simulink model "Navion_6DoF_10_auto_ascend_2023"  (R2024a)
settings: Solver=ode45  StartTime=0.0  StopTime=500  FixedStep=.01  MaxStep=.004  RelTol=1e-5  EnableMultiTasking=on
values from neighbouring files (symbols this model uses):
  ac = [0 0 0]    [Navion_Geom_temp.m]
  b = 33.4    [Navion_Geom_temp.m]
  cbar = 5.7    [Navion_Geom_temp.m]
  cda2 = 0.33    [Navion_Geom_temp.m]
  cdo = 0.05    [Navion_Geom_temp.m]
  cg = [0 0 0]    [Navion_Geom_temp.m]
  cla = 4.44    [Navion_Geom_temp.m]
  cladot = 0    [Navion_Geom_temp.m]
  clb = -0.074    [Navion_Geom_temp.m]
  clda = -0.134    [Navion_Geom_temp.m]
  clde = 0.355    [Navion_Geom_temp.m]
  cldr = 0.107    [Navion_Geom_temp.m]
  clo = 0.41    [Navion_Geom_temp.m]
  clp = -0.410    (= -0.41)    [Navion_Geom_temp.m]
  clq = 3.8    [Navion_Geom_temp.m]
  clr = 0.107    [Navion_Geom_temp.m]
  cma = -0.683    [Navion_Geom_temp.m]
  cmadot = -4.36    [Navion_Geom_temp.m]
  cmde = -0.923    [Navion_Geom_temp.m]
  cmq = -9.96    [Navion_Geom_temp.m]
  cnb = 0.071    [Navion_Geom_temp.m]
  cnda = -0.0035    [Navion_Geom_temp.m]
  cndr = -0.072    [Navion_Geom_temp.m]
  cnp = -0.0575    [Navion_Geom_temp.m]
  cnr = -0.125    [Navion_Geom_temp.m]
  cyb = -0.564    [Navion_Geom_temp.m]
  cydr = 0.157    [Navion_Geom_temp.m]
  eng = [0 0 0]    [Navion_Geom_temp.m]
  initalt = 5000    [Navion_Geom_temp.m]
  initbank = 0    [Navion_Geom_temp.m]
  initeast = 0    [Navion_Geom_temp.m]
  inithead = 0    [Navion_Geom_temp.m]
  initnorth = 0    [Navion_Geom_temp.m]
  initp = 0    [Navion_Geom_temp.m]
  initpitch = initw/initu    (= 0)    [Navion_Geom_temp.m]
  initq = 0    [Navion_Geom_temp.m]
  initr = 0    [Navion_Geom_temp.m]
  initu = 223    [Navion_Geom_temp.m]
  initv = 0    [Navion_Geom_temp.m]
  initw = 0    [Navion_Geom_temp.m]
  jx = 1048    [Navion_Geom_temp.m]
  jxz = 0    [Navion_Geom_temp.m]
  jy = 3000    [Navion_Geom_temp.m]
  jz = 3500    [Navion_Geom_temp.m]
  sw = 184    [Navion_Geom_temp.m]
  weight = 2750    [Navion_Geom_temp.m]
undefined symbols (not defined in the file or in its folder): Earth, WGS84
libraries: simulink_extras x9, slpidlib x6, aerolibfltsims x2, simulink x2, aerolibtransform2 x1, aerolibanimutils x1
(part 1 of 2)
settings Model: Creator=andersop  LastModifiedBy=kaleb
settings SolverCC: InitialStep=.004  AlgebraicLoopSolver=TrustRegion
settings DataIOCC: LimitDataPoints=on  SaveFormat=Array  SignalLoggingSaveFormat=ModelDataLogs  SaveState=on  ReturnWorkspaceOutputs=off  SignalLoggingName=sigsOut
settings OptimizationCC: ExpressionDepthLimit=2147483647  InitFltsAndDblsToZero=on  LifeSpan=inf
settings DebuggingCC: SaveWithParameterizedLinksMsg=none  UnderspecifiedInitializationDetection=Classic  MergeDetectMultiDrivingBlocksExec=none  SignalResolutionControl=TryResolveAllWithWarning  MultiTaskDSMMsg=warning  MultiTaskCondExecSysMsg=none  FcnCallInpInsideContextMsg=warning  UnconnectedInputMsg=warning  UnconnectedOutputMsg=warning  UnconnectedLineMsg=warning  StateNameClashWarn=warning  SFUnexpectedBacktrackingDiag=warning  SFNoUnconditionalDefaultTransitionDiag=warning  SFExecutionAtInitializationDiag=none  ArithmeticOperatorsInVariantConditions=warning
settings HardwareCC: ProdBitPerPointer=32  ProdBitPerSizeT=32  ProdBitPerPtrDiffT=32  ProdLargestAtomicFloat=None  ProdIntDivRoundTo=Undefined  ProdEndianess=Unspecified  ProdWordSize=32  ProdHWDeviceType=32-bit Generic  TargetUnknown=on
settings ModelReferenceCC: PropagateSignalLabelsOutOfModel=off
settings SFSimCC: SimUseLocalCustomCode=off  CustomCodeUndefinedFunction=UseInterfaceOnly
settings RTWCC: RTWUseLocalCustomCode=off  GPUComputeCapability=3.5
settings CodeAppCC: StateflowObjectComments=on
settings GRTTargetCC: TargetFcnLib=ansi_tfl_tmw.mat  TargetLangStandard=C89/C90 (ANSI)  ModelReferenceCompliant=off  CombineOutputUpdateFcns=off  MatFileLogging=off  GRTInterface=on
settings ConfigComp: CovMetricSettings=dw  CovSaveCumulativeToWorkspaceVar=on  CovSaveSingleToWorkspaceVar=on  CovExternalEMLEnable=off

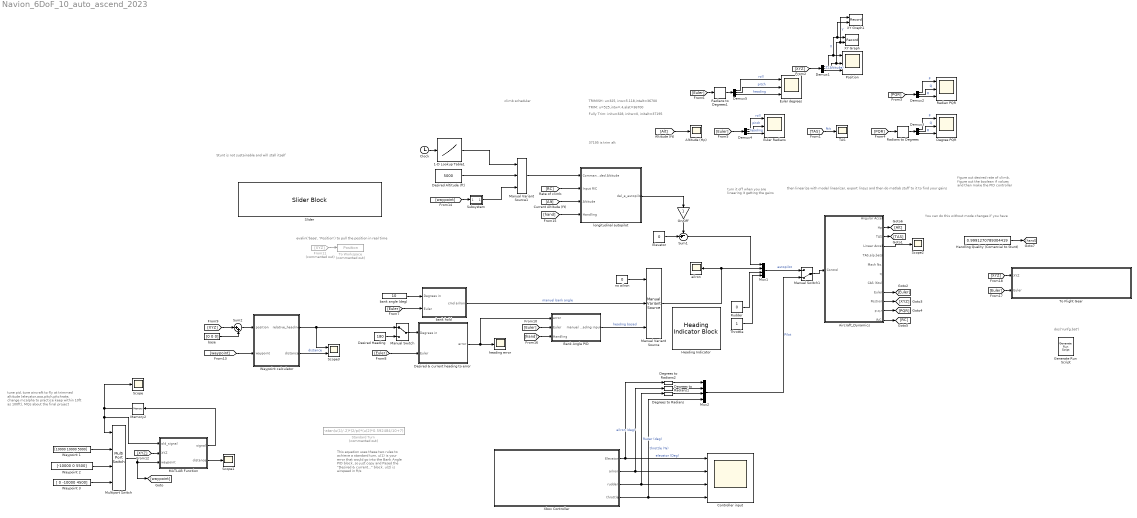
== system Navion_6DoF_10_auto_ascend_2023 ==
  note: tune pid, tune aircraft to fly at trimmed altitude (elevator,aoa,pitch,pitchrate, change mcalpha to practice keep within 10ft as 100ft), MQs about the final project
  note: Stunt is not sustainable and will stall itself
  note: This equation uses these two rules to achieve a standard turn, u(1) is your error that would go into the Bank Angle PID block, so just copy and Pased the "Desired & current..." block. u(2) is airspeed in ft/s
  note: evalin('base', 'Position') to pull the position in real time
  note: You can do this without mode changes if you have
  note: figure out desired rate of climb, figure out the boolean if values and then make the PID controller
  note: then linearize with model linearizer, export linsys and then do matlab stuff to it to find your gains
  note: turn it off when you are linearing it getting the gains
  note: climb scheduler
  note: 37195 is trim alt
  note: Fully Trim: initu=328, initw=0, initalt=37195
  note: TRIM: u=525,intw=.4,alat=36700
  note: TRIMISH: u=325, inw=5.118,intalt=36700
  note: dos('runfg.bat')
  1-D Lookup Table1 : Lookup_n-D  NumberOfTableDimensions=1  BreakpointsForDimension1=[0 50 51 400 401 800 801 900 901 1500]  Table=[37195;37195;34000;34000;37000;37000;30000;30000;31000;31000]  InternalRulePriority=Speed  RndMeth=Simplest
  Aircraft_Dynamics : Subsystem
  Altitude (Hp) : Scope
  Bank Angle PID : Subsystem
  Clock : Clock
  Controller input : Scope  NumInputPorts=4
  Degree PQR : Scope  NumInputPorts=3
  Degrees to Radians : simulink_extras/Transformations/Degrees to Radians
  Degrees to Radians1 : simulink_extras/Transformations/Degrees to Radians
  Degrees to Radians2 : simulink_extras/Transformations/Degrees to Radians
  Demux{1..5} (5 alike) : Demux  Outputs=3
  Desired & current heading to error : Subsystem
  Desired Altitude (ft) : Constant  Value=5000
  Desired Heading : Constant  Value=180
  Elevator : Constant  Value=0
  Euler Radians : Scope  NumInputPorts=3
  Euler degrees : Scope  NumInputPorts=3
  From11 : From  Commented=on  GotoTag=XYZ
  Generate Run Script : aerolibfltsims/Generate Run Script  Architecture=Win64  dataFlow=Send  GeometryModelName=c172p  AirportId=KSFO  RunwayId=01L  InitialAltitude=0  InitialHeading=0  OffsetDistance=0  OffsetAzimuth=0  InstallScenery=off  DisableShaders=on  OriginAddress=127.0.0.1  DestinationPort=5502  OriginPort=5505  LocalAddress=127.0.0.1  OutputFileName=runfg.bat  FlightGearBaseDirectory=C:\Program Files\FlightGear 2020.3
  Handling Quality (Comercial to Stunt) : Constant  Value=0.9991270789304419
  Heading Indicator : HeadingIndicatorBlock
  MATLAB Function : MATLAB Function  TreatAsAtomicUnit=on
  Manual Variant Source : simulink/Signal Routing/Manual Variant Source  NumChoices=3  LabelModeActiveChoice=V_3
  Manual Variant Source1 : simulink/Signal Routing/Manual Variant Source  NumChoices=3  LabelModeActiveChoice=V_3
  Manual Switch : ManualSwitch
  Manual Switch1 : ManualSwitch  CurrentSetting=0
  Memory2 : Memory  InitialCondition=1
  Multiport Switch : MultiPortSwitch  SaturateOnIntegerOverflow=off  InputSameDT=off
  Mux1 : Mux
  Mux2 : Mux
  On/Off : Gain
  Position : Scope  NumInputPorts=3
  Radian PQR : Scope  NumInputPorts=3
  Radians to Degrees : simulink_extras/Transformations/Radians to Degrees
  Radians to Degrees1 : simulink_extras/Transformations/Radians to Degrees
  Rudder : Constant  Value=0
  Scope : Scope
  Scope1 : Scope
  Scope2 : Scope
  Scope3 : Scope  NumInputPorts=2
  Slider : SliderBlock  ScaleMax=1
  Standard Turn : Fcn  Commented=on  Expr=-atan(u(1)/.2)*(2/pi)*(u(2)*0.592484/10+7)
  Subsystem : Subsystem
  Sum1 : Sum  Inputs=-+|
  Sum2 : Sum  Inputs=|++
  TAS : Scope
  Throttle : Constant
  To Flight Gear : Subsystem
  To Workspace : ToWorkspace  Commented=on  VariableName=Position  SaveFormat=Timeseries  SampleTime=-1
  Waypoint 1 : Constant  Value=[10000 10000 5000]
  Waypoint 2 : Constant  Value=[-10000 0 5500]
  Waypoint 3 : Constant  Value=[ 0 -10000 4500]
  Waypoint calculator : MATLAB Function  TreatAsAtomicUnit=on
  XY Graph : Record  FileSettingsInternal="{\"entries\":[{\"content\":{\"excelSettings\":{\"content\":{},\"type\":\"Streamout.ExcelSettings\"}},\"type\":\"Streamout.FileSettingStorage\",\"uuid\":\"\"}],\"packageUris\":[\"http:\\/\\/schema.mathworks.com\\/mf0\\/streamout_blocks\\/R2020a\"],\"version\":\"1.0\"}"  Layout=[1 1]  SignalsInternal="{\"entries\":[{\"content\":{\"signals\":[{\"content\":{\"blockPath\":[],\"dimensions\":[1],\"domain\":\"\",\"lineColor\":\"#a2142f\",\"lineWidth\":2,\"port\":1,\"sid\":[\"\"],\"signalID\":1,\"signalName\":\"X\"},\"type\":\"RecordBlkView.Signal\",\"uuid\":\"\"},{\"content\":{\"blockPath\":[],\"dimensions\":[1],\"domain\":\"\",\"lineColor\":\"#139fff\",\"lineWidth\":2,\"port\":2,\"sid\":[\"\"],\"signalID\":2,\"signalName\":\"Y\"},\"type\":\"RecordBlkView.Signal\",\"uuid\":\"\"}]},\"type\":\"RecordBlkView.InputSignals\",\"uuid\":\"\"}],\"packageUris\":[\"http:\\/\\/schema.mathworks.com\\/mf0\\/streamout_blocks\\/R2020a\"],\"version\":\"1.0\"}"  VisualizationBindings="{\"sparklinesplugin\":{\"info\":[{\"bindingParametersList\":[],\"subplotID\":1}]}}"  CompatibilityTag=XY
  XY Graph1 : Record  FileSettingsInternal="{\"entries\":[{\"content\":{\"excelSettings\":{\"content\":{},\"type\":\"Streamout.ExcelSettings\"}},\"type\":\"Streamout.FileSettingStorage\",\"uuid\":\"\"}],\"packageUris\":[\"http:\\/\\/schema.mathworks.com\\/mf0\\/streamout_blocks\\/R2020a\"],\"version\":\"1.0\"}"  Layout=[1 1]  SignalsInternal="{\"entries\":[{\"content\":{\"signals\":[{\"content\":{\"blockPath\":[],\"dimensions\":[1],\"domain\":\"\",\"lineColor\":\"#a2142f\",\"plots\":[ 1 ],\"port\":1,\"sid\":[\"\"],\"signalID\":1,\"signalName\":\"Y\"},\"type\":\"RecordBlkView.Signal\",\"uuid\":\"\"},{\"content\":{\"blockPath\":[],\"dimensions\":[1],\"domain\":\"\",\"lineColor\":\"#139fff\",\"plots\":[ 1 ],\"port\":2,\"sid\":[\"\"],\"signalID\":2,\"signalName\":\"X\"},\"type\":\"RecordBlkView.Signal\",\"uuid\":\"\"}]},\"type\":\"RecordBlkView.InputSignals\",\"uuid\":\"\"}],\"packageUris\":[\"http:\\/\\/schema.mathworks.com\\/mf0\\/streamout_blocks\\/R2020a\"],\"version\":\"1.0\"}"  VisualizationBindings="{\"xyplotplugin\":{\"info\":[{\"series\":[{\"bindingParametersList\":[{\"parameter\":\"X-Axis\",\"signalID\":1,\"signalName\":\"Y\"},{\"parameter\":\"Y-Axis\",\"signalID\":2,\"signalName\":\"X\"}],\"seriesID\":0}],\"subplotID\":1}]}}"  CompatibilityTag=XY
  Xbox Controller : Subsystem
  ailron : Scope
  bank angle (deg) : Constant  Value=10
  bank hold : Subsystem
  base : Constant  Value=[0 0 0]
  heading error : Scope
  longitudinal autopilot : Subsystem
  no ailron : Constant  Value=0
  wires:
  Elevator/1 -> Sum1/2
  Throttle/1 -> Mux1/4
  Mux1/1 -> Manual Switch1/1  "autopilot"
  Aircraft_Dynamics/2(Hp) -> [Alt]
  Aircraft_Dynamics/3(TAS) -> [TAS]
  Aircraft_Dynamics/9(Euler) -> [Euler]
  Aircraft_Dynamics/10(Postion) -> [XYZ]
  Aircraft_Dynamics/11(p,q,r) -> [PQR]
  [TAS] -> TAS/1  "ft/s"
  Demux1/3 -> Position/3  "Z (Altitude)"
  Demux1/2 -> XY Graph1/1, XY Graph/2, Position/2  "Y"
  Demux1/1 -> XY Graph1/2, XY Graph/1, Position/1  "X"
  [XYZ] -> Demux1/1
  [PQR] -> Demux2/1
  Demux2/1 -> Radian PQR/1  "P"
  Demux2/2 -> Radian PQR/2  "Q"
  Demux2/3 -> Radian PQR/3  "R"
  Demux3/3 -> Degree PQR/3  "R"
  Demux3/2 -> Degree PQR/2  "Q"
  Demux3/1 -> Degree PQR/1  "P"
  [PQR] -> Radians to Degrees/1
  Radians to Degrees/1 -> Demux3/1
  [Euler] -> Demux4/1
  Demux4/1 -> Euler Radians/1  "roll"
  Demux4/2 -> Euler Radians/2  "pitch"
  Demux4/3 -> Euler Radians/3  "heading"
  Demux5/3 -> Euler degrees/3  "heading"
  Demux5/2 -> Euler degrees/2  "pitch"
  Demux5/1 -> Euler degrees/1  "roll"
  [Euler] -> Radians to Degrees1/1
  Radians to Degrees1/1 -> Demux5/1
  Sum1/1 -> Mux1/1
  On/Off/1 -> Sum1/1
  [Alt] -> Altitude (Hp)/1
  longitudinal autopilot/1(del_e_autopilot) -> On/Off/1
  Desired Altitude (ft)/1 -> Manual Variant Source1/2
  [Alt] -> longitudinal autopilot/3(Altitude)
  Aircraft_Dynamics/12(R/C) -> [RC]
  [RC] -> longitudinal autopilot/2(Input R/C)
  Clock/1 -> 1-D Lookup Table1/1
  Rudder/1 -> Mux1/3
  [XYZ] -> Sum2/1
  Waypoint calculator/2(distance) -> Scope3/2  "distance"
  Waypoint calculator/1(relative_heading) -> Manual Switch/1, Scope3/1
  Desired Heading/1 -> Manual Switch/2
  Manual Variant Source/1 -> Mux1/2, ailron/1
  bank angle (deg)/1 -> bank hold/1(Degrees in)
  bank hold/1(cmd ailron) -> Manual Variant Source/2  "manuel bank angle"
  no ailron/1 -> Manual Variant Source/1
  [Euler] -> Desired & current heading to error/2(Euler)
  [Euler] -> bank hold/2(Euler)
  Desired & current heading to error/1(error) -> Bank Angle PID/1(error), heading error/1
  [Euler] -> Bank Angle PID/2(Euler)
  Bank Angle PID/1(manuel heading input) -> Manual Variant Source/3  "heading based"
  Waypoint 1/1 -> Multiport Switch/2
  Waypoint 2/1 -> Multiport Switch/3
  Waypoint 3/1 -> Multiport Switch/4
  Sum2/1 -> Waypoint calculator/1(position)
  base/1 -> Sum2/2
  From11/1 -> To Workspace/1
  Manual Switch/1 -> Desired & current heading to error/1(Degrees in)
  Multiport Switch/1 -> [waypoint], MATLAB Function/3(waypoint)
  [XYZ] -> MATLAB Function/2(XYZ)
  MATLAB Function/1(signal) -> Memory2/1
  Memory2/1 -> Multiport Switch/1, MATLAB Function/1(old_signal), Scope/1
  [waypoint] -> Waypoint calculator/2(waypoint)
  Manual Variant Source1/1 -> longitudinal autopilot/1(Commanded Altitude)
  1-D Lookup Table1/1 -> Manual Variant Source1/1
  [waypoint] -> Subsystem/1(In1)
  Subsystem/1(Out1) -> Manual Variant Source1/3
  MATLAB Function/2(distance) -> Scope1/1
  Aircraft_Dynamics/4(Linear Accel) -> Scope2/1
  Handling Quality (Comercial to Stunt)/1 -> [hand]
  [hand] -> longitudinal autopilot/4(Handling)
  [hand] -> Bank Angle PID/3(Handling)
  Xbox Controller/2(ailron) -> Degrees to Radians1/1, Controller input/2  "ailron (deg)"
  Xbox Controller/1(Elevator) -> Degrees to Radians2/1, Controller input/1  "elevator (Deg)"
  Xbox Controller/3(rudder) -> Degrees to Radians/1, Controller input/3  "Ruder (deg)"
  Xbox Controller/4(throttle) -> Mux2/4, Controller input/4  "throttle (%)"
  Degrees to Radians/1 -> Mux2/3
  Degrees to Radians2/1 -> Mux2/1
  Degrees to Radians1/1 -> Mux2/2
  Manual Switch1/1 -> Aircraft_Dynamics/1(Control)
  Mux2/1 -> Manual Switch1/2  "Pilot"
  [XYZ] -> To Flight Gear/1(XYZ)
  [Euler] -> To Flight Gear/2(Euler)

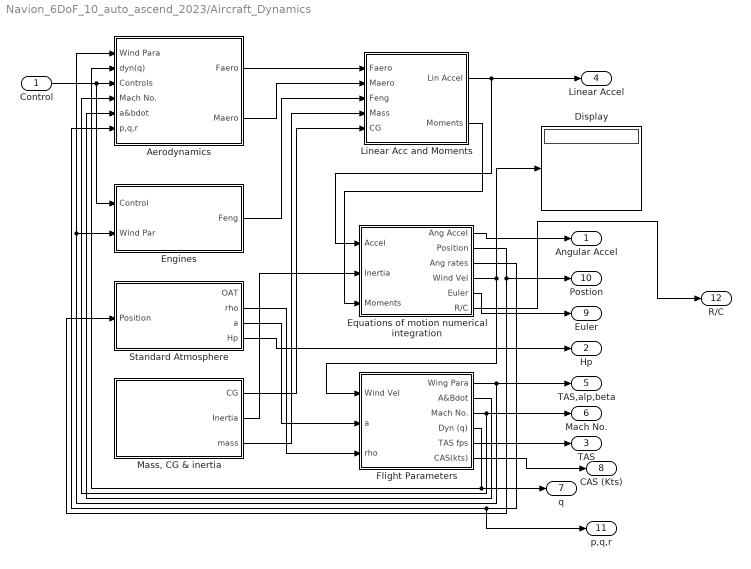
== system Navion_6DoF_10_auto_ascend_2023/Aircraft_Dynamics ==
  Control : Inport
  Aerodynamics : Subsystem
  Display : Display
  Engines : Subsystem
  "Equations of motion numerical integration " : Subsystem
  Flight Parameters : Subsystem
  Linear Acc and Moments : Subsystem
  "Mass, CG & inertia" : Subsystem
  Standard Atmosphere : Subsystem
  Angular Accel : Outport
  Hp : Outport  Port=2
  TAS : Outport  Port=3
  Linear Accel : Outport  Port=4
  TAS,alp,beta : Outport  Port=5
  Mach No. : Outport  Port=6
  q : Outport  Port=7
  CAS (Kts) : Outport  Port=8
  Euler : Outport  Port=9
  Postion : Outport  Port=10
  p,q,r : Outport  Port=11
  R/C : Outport  Port=12
  wires:
  Aerodynamics/1(Faero) -> Linear Acc and Moments/1(Faero)
  Aerodynamics/2(Maero) -> Linear Acc and Moments/2(Maero)
  Control/1 -> Aerodynamics/3(Controls), Engines/1(Control)
  Engines/1(Feng) -> Linear Acc and Moments/3(Feng)
  "Mass, CG & inertia"/1(CG) -> Linear Acc and Moments/5(CG)
  "Mass, CG & inertia"/2(Inertia) -> "Equations of motion numerical integration "/2(Inertia)
  Linear Acc and Moments/1(Lin Accel) -> "Equations of motion numerical integration "/1(Accel), Linear Accel/1
  Linear Acc and Moments/2(Moments) -> "Equations of motion numerical integration "/3(Moments)
  "Equations of motion numerical integration "/3(Ang rates) -> Aerodynamics/6(p,q,r), p,q,r/1
  "Equations of motion numerical integration "/4(Wind Vel) -> Flight Parameters/1(Wind Vel), Display/1
  Flight Parameters/1(Wing Para) -> TAS,alp,beta/1, Aerodynamics/1(Wind Para), Engines/2(Wind Par)
  Flight Parameters/4(Dyn (q)) -> Aerodynamics/2(dyn(q)), q/1
  Flight Parameters/3(Mach No.) -> Mach No./1, Aerodynamics/4(Mach No.)
  Flight Parameters/2(A&Bdot) -> Aerodynamics/5(a&bdot)
  "Equations of motion numerical integration "/2(Position) -> Postion/1, Standard Atmosphere/1(Position)
  "Equations of motion numerical integration "/1(Ang Accel) -> Angular Accel/1
  Standard Atmosphere/4(Hp) -> Hp/1
  Flight Parameters/5(TAS fps) -> TAS/1
  Flight Parameters/6(CAS(kts)) -> CAS (Kts)/1
  "Equations of motion numerical integration "/5(Euler) -> Euler/1
  Standard Atmosphere/3(a) -> Flight Parameters/2(a)
  Standard Atmosphere/2(rho) -> Flight Parameters/3(rho)
  "Mass, CG & inertia"/3(mass) -> Linear Acc and Moments/4(Mass)
  "Equations of motion numerical integration "/6(R/C) -> R/C/1

== system Navion_6DoF_10_auto_ascend_2023/Bank Angle PID ==
  note: agressive, will make it
  note: safe, wont make it
  note: was 50/23
  error : Inport
  Euler : Inport  Port=2
  Handling : Inport  Port=3
  Mux : Mux  Inputs=2
  PID Controller : slpidlib/PID Controller  Controller=PID  Form=Parallel  TimeDomain=Continuous-time  UseExternalTs=off  SampleTime=-1  IntegratorMethod=Forward Euler  FilterMethod=Forward Euler  ControllerParametersSource=internal  P=-0.426657604109643  I=-0.0814157073414658  UseKiTs=off  D=0.00186667465731567  UseExternalDerivativeSource=off  N=228.565595208321  UseFilter=on  TunerSelectOption=Transfer Function Based (PID Tuner App)  InitialConditionSource=internal  InitialConditionForIntegrator=0  InitialConditionForFilter=0  DifferentiatorICPrevScaledInput=0  ExternalReset=none  TrackingMode=off  Kt=1  LimitOutput=on  SatLimitsSource=internal  UpperSaturationLimit=.5  LowerSaturationLimit=-.5  LinearizeAsGain=off  AntiWindupMode=none  Kb=1  LimitIntegrator=off  UpperIntegratorSaturationLimit=inf  LowerIntegratorSaturationLimit=-inf  POutMin=[]  POutMax=[]  IOutMin=[]  IOutMax=[]  DOutMin=[]  DOutMax=[]  NOutMin=[]  NOutMax=[]  SumOutMin=[]  SumOutMax=[]  SaturationOutMin=[]  SaturationOutMax=[]  PParamMin=[]  PParamMax=[]  IParamMin=[]  IParamMax=[]  DParamMin=[]  DParamMax=[]  NParamMin=[]  NParamMax=[]  KbParamMin=[]  KbParamMax=[]  KtParamMin=[]  KtParamMax=[]  KbOutMin=[]  KbOutMax=[]  KtOutMin=[]  KtOutMax=[]  IntegratorOutMin=[]  IntegratorOutMax=[]  FilterOutMin=[]  FilterOutMax=[]  SumI1OutMin=[]  SumI1OutMax=[]  SumI2OutMin=[]  SumI2OutMax=[]  SumI3OutMin=[]  SumI3OutMax=[]  SumI4OutMin=[]  SumI4OutMax=[]  SumDOutMin=[]  SumDOutMax=[]  DifferentiatorOutMin=[]  DifferentiatorOutMax=[]  FilterDiffOutCoefMin=[]  FilterDiffOutCoefMax=[]  ReciprocalOutMin=[]  ReciprocalOutMax=[]  SumDenOutMin=[]  SumDenOutMax=[]  SumNumOutMin=[]  SumNumOutMax=[]  DivideOutMin=[]  DivideOutMax=[]  UdiffTsProdOutMin=[]  UdiffTsProdOutMax=[]  NTsProdOutMin=[]  NTsProdOutMax=[]  UintegralTsProdOutMin=[]  UintegralTsProdOutMax=[]  UngainTsProdOutMin=[]  UngainTsProdOutMax=[]  ClampingZeroOutDataTypeStr=Inherit: Inherit via back propagation  ClampingZeroOutMin=[]  ClampingZeroOutMax=[]  FilterDenConstantOutDataTypeStr=Inherit: Inherit via back propagation  FilterDenConstantOutMin=[]  FilterDenConstantOutMax=[]  PCopyOutDataTypeStr=Inherit: Inherit via back propagation  PCopyOutMin=[]  PCopyOutMax=[]  NCopyOutDataTypeStr=Inherit: Inherit via back propagation  NCopyOutMin=[]  NCopyOutMax=[]  IntegratorContinuousStateAttributes=''  IntegratorStateMustResolveToSignalObject=off  IntegratorRTWStateStorageClass=Auto  FilterContinuousStateAttributes=''  FilterStateMustResolveToSignalObject=off  FilterRTWStateStorageClass=Auto  ParallelPVariant=InternalParameters  IdealPVariant=Disabled  IVariant=InternalParameters  DVariant=InternalParameters  IntegratorVariant=Continuous  SatVariant=Enabled  AWVariant=Passthrough  PCopyVariant=Disabled  TRVariant=Disabled  FdbkBlocksVariant=Forward  IdealPFdbkVariant=Disabled  SatFdbkVariant=Disabled  DerivativeFilterVariant=ContFilter  NVariant=InternalParameters  NCopyVariant=Disabled  FilterICVariant=InternalICsFilter  IntegratorICVariant=InternalICs  ExternalResetVariant=Disabled  TRSumVariant=Passthrough  SumFdbkVariant=Disabled  SumVariant=Sum_PID  TsampFilterVariant=InternalTs  TsampNgainVariant=Passthrough  TsampIntegralVariant=Disabled_SignalSpec  ExternalSaturationOutDataTypeStr=Inherit: Same as second input  DerivativeSourceVariant=ErrorSignal
  Radians to Degrees3 : simulink_extras/Transformations/Radians to Degrees
  Sum2 : Sum  Inputs=|+-
  heading error to bank angle2 : Fcn  Commented=on  Expr=-(atan(u(1)/50)*23)
  heading error to bank angle3 : Fcn  Commented=on  Expr=-(atan(u(1)/15)*23)
  heading error to bank angle4 : Fcn  Expr=-(atan(u(1)/(-35*u(2)+50))*23)
  roll : Subsystem
  manuel heading input : Outport
  wires:
  Euler/1 -> roll/1(In1)
  roll/1(Out1) -> Radians to Degrees3/1
  Sum2/1 -> PID Controller/1
  error/1 -> Mux/1
  PID Controller/1 -> manuel heading input/1  "manuel heading input"
  Radians to Degrees3/1 -> Sum2/2
  Mux/1 -> heading error to bank angle4/1
  Handling/1 -> Mux/2
  heading error to bank angle3/1 -> ?
  heading error to bank angle4/1 -> Sum2/1

== system Navion_6DoF_10_auto_ascend_2023/Desired & current heading to error ==
  Degrees in : Inport
  Euler : Inport  Port=2
  Degrees to Radians1 : simulink_extras/Transformations/Degrees to Radians
  Demux6 : Demux  Outputs=3
  MATLAB Function : MATLAB Function  TreatAsAtomicUnit=on
  Radians to Degrees2 : simulink_extras/Transformations/Radians to Degrees
  Scope : Scope
  Terminator2 : Terminator
  Terminator3 : Terminator
  error : Outport
  wires:
  Demux6/2 -> Terminator2/1
  Euler/1 -> Scope/1, Demux6/1
  Degrees in/1 -> Degrees to Radians1/1
  Demux6/1 -> Terminator3/1
  Demux6/3 -> MATLAB Function/1(heading)  "headin"
  MATLAB Function/1(error) -> Radians to Degrees2/1
  Degrees to Radians1/1 -> MATLAB Function/2(desired)  "command heading"
  Radians to Degrees2/1 -> error/1

== system Navion_6DoF_10_auto_ascend_2023/Subsystem ==
  In1 : Inport
  Demux : Demux  Outputs=3
  Terminator : Terminator
  Terminator1 : Terminator
  Out1 : Outport
  wires:
  Demux/1 -> Terminator/1
  Demux/2 -> Terminator1/1
  Demux/3 -> Out1/1
  In1/1 -> Demux/1

== system Navion_6DoF_10_auto_ascend_2023/To Flight Gear ==
  XYZ : Inport
  Euler : Inport  Port=2
  Constant8 : Constant  Value=0
  Demux : Demux  Outputs=3
  Demux6 : Demux  Outputs=2
  Flat Earth to LLA : aerolibtransform2/Flat Earth to LLA  units=English  ptype=Earth (WGS84)  F=1/298.257223563  R=20925646.3255  refPosPort=off  LL0=[37.60787906487077, -122.38296272343536]  psi=0
  FlightGear Preconfigured 6DoF Animation : aerolibfltsims/FlightGear Preconfigured 6DoF Animation  xFlightGearVersion=v2019.1  DestinationIpAddress=127.0.0.1  DestinationPort=5502  SampleTime=1/30  packetVersion=24
  Gain1 : Gain  Gain=-1
  Mux : Mux  Inputs=3
  Mux4 : Mux
  wires:
  Demux6/2 -> Mux4/1
  Constant8/1 -> Flat Earth to LLA/2
  Mux4/1 -> FlightGear Preconfigured 6DoF Animation/1
  Euler/1 -> Mux4/4
  Gain1/1 -> Mux/3
  Demux/1 -> Mux/1
  Demux/3 -> Gain1/1
  Mux/1 -> Flat Earth to LLA/1
  Demux6/1 -> Mux4/2
  Flat Earth to LLA/2 -> Mux4/3
  Flat Earth to LLA/1 -> Demux6/1
  Demux/2 -> Mux/2
  XYZ/1 -> Demux/1

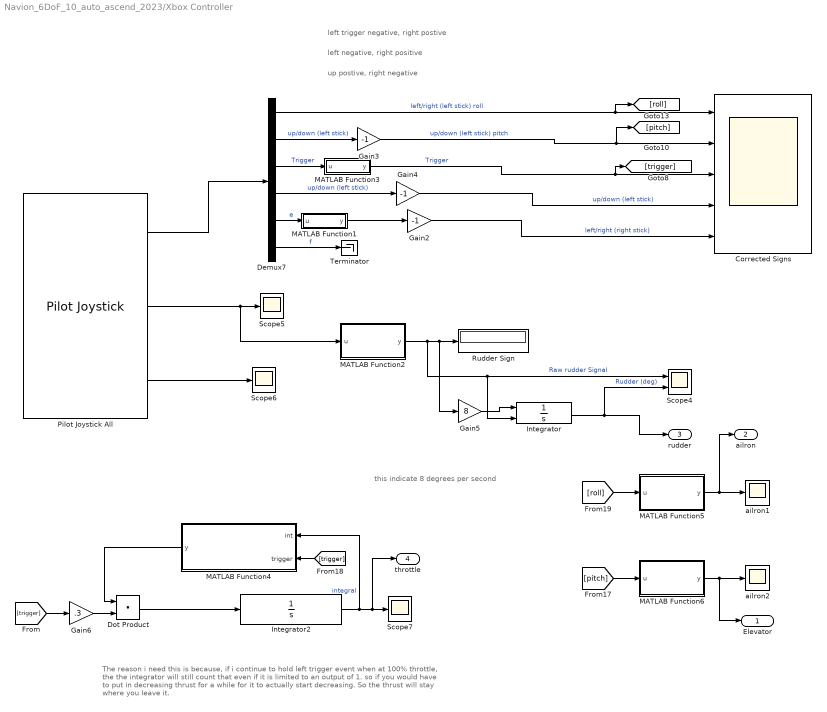
== system Navion_6DoF_10_auto_ascend_2023/Xbox Controller ==
  note: The reason i need this is because, if i continue to hold left trigger event when at 100% throttle, the the integrator will still count that even if it is limited to an output of 1. so if you would have to put in decreasing thrust for a while for it to actually start decreasing. So the thrust will stay where you leave it.
  note: left trigger negative, right postive
  note: left negative, right positive
  note: this indicate 8 degrees per second
  note: up postive, right negative
  Corrected Signs : Scope  NumInputPorts=5
  Demux7 : Demux  Outputs=6
  Dot Product : DotProduct  OutDataTypeStr=Inherit: Inherit via internal rule
  Gain2 : Gain  Gain=-1
  Gain3 : Gain  Gain=-1
  Gain4 : Gain  Gain=-1
  Gain5 : Gain  Gain=8
  Gain6 : Gain  Gain=.3
  Integrator : Integrator  ExternalReset=either  LimitOutput=on  UpperSaturationLimit=30  LowerSaturationLimit=-30
  Integrator2 : Integrator  LimitOutput=on  UpperSaturationLimit=1  LowerSaturationLimit=0
  MATLAB Function1 : MATLAB Function  TreatAsAtomicUnit=on
  MATLAB Function2 : MATLAB Function  TreatAsAtomicUnit=on
  MATLAB Function3 : MATLAB Function  TreatAsAtomicUnit=on
  MATLAB Function4 : MATLAB Function  TreatAsAtomicUnit=on
  MATLAB Function5 : MATLAB Function  TreatAsAtomicUnit=on
  MATLAB Function6 : MATLAB Function  TreatAsAtomicUnit=on
  Pilot Joystick All : aerolibanimutils/Pilot Joystick  JoystickID=Joystick1  OutputConfiguration=AllOutputs  SampleTime=1/30
      settings: LibrarySourceBlock=aerolibanimutils/Pilot Joystick All
  Rudder Sign : Display
  Scope4 : Scope  NumInputPorts=2
  Scope5 : Scope
  Scope6 : Scope
  Scope7 : Scope
  Terminator : Terminator
  ailron1 : Scope
  ailron2 : Scope
  Elevator : Outport
  ailron : Outport  Port=2
  rudder : Outport  Port=3
  throttle : Outport  Port=4
  wires:
  Pilot Joystick All/3 -> Scope6/1
  Demux7/1 -> [roll], Corrected Signs/1  "left/right (left stick) roll"
  MATLAB Function6/1(y) -> Elevator/1, ailron2/1
  Gain4/1 -> Corrected Signs/4  "up/down (left stick)"
  MATLAB Function4/1(y) -> Dot Product/1
  MATLAB Function5/1(y) -> ailron/1, ailron1/1
  MATLAB Function2/1(y) -> Integrator/2, Scope4/1, Gain5/1, Rudder Sign/1  "Raw rudder Signal"
  Pilot Joystick All/2 -> MATLAB Function2/1(u), Scope5/1
  MATLAB Function3/1(y) -> [trigger], Corrected Signs/3  "Trigger"
  Integrator2/1 -> MATLAB Function4/1(int), throttle/1, Scope7/1  "integral"
  Gain2/1 -> Corrected Signs/5  "left/right (right stick)"
  Demux7/4 -> Gain4/1  "up/down (left stick)"
  [roll] -> MATLAB Function5/1(u)
  Demux7/6 -> Terminator/1  "f"
  Gain3/1 -> [pitch], Corrected Signs/2  "up/down (left stick) pitch"
  Pilot Joystick All/1 -> Demux7/1
  Integrator/1 -> Scope4/2, rudder/1  "Rudder (deg)"
  Demux7/3 -> MATLAB Function3/1(u)  "Trigger"
  Gain6/1 -> Dot Product/2
  [trigger] -> MATLAB Function4/2(trigger)
  Demux7/5 -> MATLAB Function1/1(u)  "e"
  Dot Product/1 -> Integrator2/1
  Gain5/1 -> Integrator/1
  Demux7/2 -> Gain3/1  "up/down (left stick)"
  [trigger] -> Gain6/1
  MATLAB Function1/1(y) -> Gain2/1
  [pitch] -> MATLAB Function6/1(u)

== system Navion_6DoF_10_auto_ascend_2023/bank hold ==
  Degrees in : Inport
  Euler : Inport  Port=2
  Degrees to Radians : simulink_extras/Transformations/Degrees to Radians
  Demux : Demux  Outputs=3
  PID Controller1 : slpidlib/PID Controller  Controller=PID  Form=Parallel  TimeDomain=Continuous-time  UseExternalTs=off  SampleTime=-1  IntegratorMethod=Forward Euler  FilterMethod=Forward Euler  ControllerParametersSource=internal  P=-7.93123701373715  I=-3.48374145916555  UseKiTs=off  D=-2.00987576803133  UseExternalDerivativeSource=off  N=6575.83779362094  UseFilter=on  TunerSelectOption=Transfer Function Based (PID Tuner App)  InitialConditionSource=internal  InitialConditionForIntegrator=0  InitialConditionForFilter=0  DifferentiatorICPrevScaledInput=0  ExternalReset=none  TrackingMode=off  Kt=1  LimitOutput=on  SatLimitsSource=internal  UpperSaturationLimit=.4363  LowerSaturationLimit=-.4363  LinearizeAsGain=off  AntiWindupMode=none  Kb=1  LimitIntegrator=off  UpperIntegratorSaturationLimit=inf  LowerIntegratorSaturationLimit=-inf  POutMin=[]  POutMax=[]  IOutMin=[]  IOutMax=[]  DOutMin=[]  DOutMax=[]  NOutMin=[]  NOutMax=[]  SumOutMin=[]  SumOutMax=[]  SaturationOutMin=[]  SaturationOutMax=[]  PParamMin=[]  PParamMax=[]  IParamMin=[]  IParamMax=[]  DParamMin=[]  DParamMax=[]  NParamMin=[]  NParamMax=[]  KbParamMin=[]  KbParamMax=[]  KtParamMin=[]  KtParamMax=[]  KbOutMin=[]  KbOutMax=[]  KtOutMin=[]  KtOutMax=[]  IntegratorOutMin=[]  IntegratorOutMax=[]  FilterOutMin=[]  FilterOutMax=[]  SumI1OutMin=[]  SumI1OutMax=[]  SumI2OutMin=[]  SumI2OutMax=[]  SumI3OutMin=[]  SumI3OutMax=[]  SumI4OutMin=[]  SumI4OutMax=[]  SumDOutMin=[]  SumDOutMax=[]  DifferentiatorOutMin=[]  DifferentiatorOutMax=[]  FilterDiffOutCoefMin=[]  FilterDiffOutCoefMax=[]  ReciprocalOutMin=[]  ReciprocalOutMax=[]  SumDenOutMin=[]  SumDenOutMax=[]  SumNumOutMin=[]  SumNumOutMax=[]  DivideOutMin=[]  DivideOutMax=[]  UdiffTsProdOutMin=[]  UdiffTsProdOutMax=[]  NTsProdOutMin=[]  NTsProdOutMax=[]  UintegralTsProdOutMin=[]  UintegralTsProdOutMax=[]  UngainTsProdOutMin=[]  UngainTsProdOutMax=[]  ClampingZeroOutDataTypeStr=Inherit: Inherit via back propagation  ClampingZeroOutMin=[]  ClampingZeroOutMax=[]  FilterDenConstantOutDataTypeStr=Inherit: Inherit via back propagation  FilterDenConstantOutMin=[]  FilterDenConstantOutMax=[]  PCopyOutDataTypeStr=Inherit: Inherit via back propagation  PCopyOutMin=[]  PCopyOutMax=[]  NCopyOutDataTypeStr=Inherit: Inherit via back propagation  NCopyOutMin=[]  NCopyOutMax=[]  IntegratorContinuousStateAttributes=''  IntegratorStateMustResolveToSignalObject=off  IntegratorRTWStateStorageClass=Auto  FilterContinuousStateAttributes=''  FilterStateMustResolveToSignalObject=off  FilterRTWStateStorageClass=Auto  ParallelPVariant=InternalParameters  IdealPVariant=Disabled  IVariant=InternalParameters  DVariant=InternalParameters  IntegratorVariant=Continuous  SatVariant=Enabled  AWVariant=Passthrough  PCopyVariant=Disabled  TRVariant=Disabled  FdbkBlocksVariant=Forward  IdealPFdbkVariant=Disabled  SatFdbkVariant=Disabled  DerivativeFilterVariant=ContFilter  NVariant=InternalParameters  NCopyVariant=Disabled  FilterICVariant=InternalICsFilter  IntegratorICVariant=InternalICs  ExternalResetVariant=Disabled  TRSumVariant=Passthrough  SumFdbkVariant=Disabled  SumVariant=Sum_PID  TsampFilterVariant=InternalTs  TsampNgainVariant=Passthrough  TsampIntegralVariant=Disabled_SignalSpec  ExternalSaturationOutDataTypeStr=Inherit: Same as second input  DerivativeSourceVariant=ErrorSignal
  Sum2 : Sum  Inputs=|+-
  Terminator : Terminator
  Terminator1 : Terminator
  cmd ailron : Outport
  wires:
  Euler/1 -> Demux/1
  PID Controller1/1 -> cmd ailron/1
  Demux/2 -> Terminator/1
  Demux/3 -> Terminator1/1
  Degrees to Radians/1 -> Sum2/1
  Demux/1 -> Sum2/2
  Sum2/1 -> PID Controller1/1
  Degrees in/1 -> Degrees to Radians/1

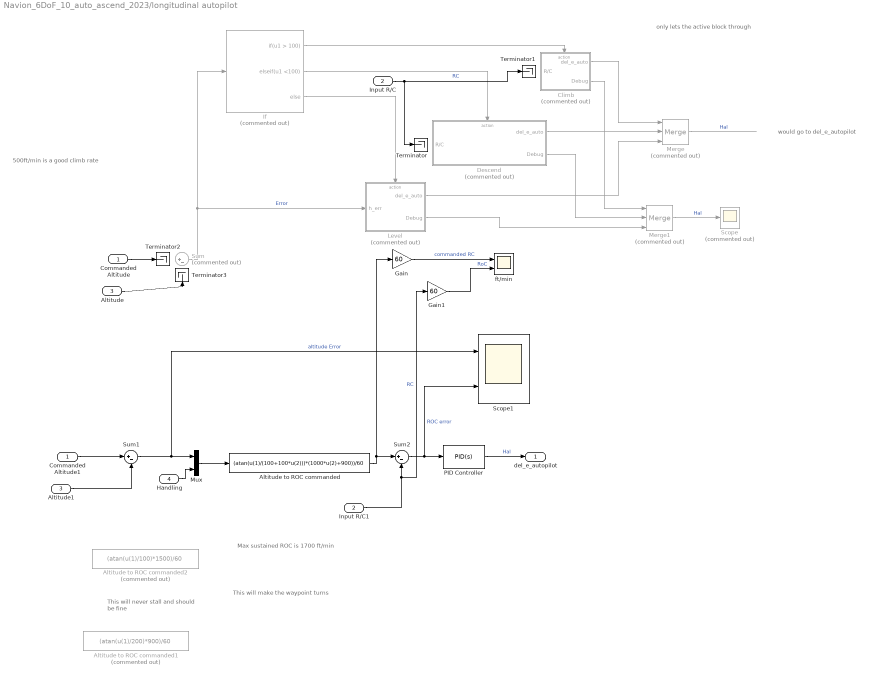
== system Navion_6DoF_10_auto_ascend_2023/longitudinal autopilot ==
  note: This will make the waypoint turns
  note: This will never stall and should be fine
  note: Max sustained ROC is 1700 ft/min
  note: would go to del_e_autopilot
  note: only lets the active block through
  note: 500ft/min is a good climb rate
  Commanded Altitude : Inport
  Input R/C : Inport  Port=2
  Altitude : Inport  Port=3
  Handling : Inport  Port=4
  Altitude to ROC commanded : Fcn  Expr=(atan(u(1)/(100+100*u(2)))*(1000*u(2)+900))/60
  Altitude to ROC commanded1 : Fcn  Commented=on  Expr=(atan(u(1)/200)*900)/60
  Altitude to ROC commanded2 : Fcn  Commented=on  Expr=(atan(u(1)/100)*1500)/60
  Altitude1 : InportShadow  Port=3
  Climb : Subsystem  Commented=on  TreatAsAtomicUnit=on
  Commanded Altitude1 : InportShadow
  Descend : Subsystem  Commented=on  TreatAsAtomicUnit=on
  Gain : Gain  Gain=60
  Gain1 : Gain  Gain=60
  If : If  Commented=on  IfExpression=u1 > 100  ElseIfExpressions=u1 <100
  Input R/C1 : InportShadow  Port=2
  Level : Subsystem  Commented=on  TreatAsAtomicUnit=on
  Merge : Merge  Commented=on  Inputs=3
  Merge1 : Merge  Commented=on  Inputs=3
  Mux : Mux  Inputs=2
  PID Controller : slpidlib/PID Controller  Controller=PID  Form=Parallel  TimeDomain=Continuous-time  UseExternalTs=off  SampleTime=-1  IntegratorMethod=Forward Euler  FilterMethod=Forward Euler  ControllerParametersSource=internal  P=0.00283704832127686  I=0.000685314377920621  UseKiTs=off  D=0.00128849134069854  UseExternalDerivativeSource=off  N=331.162272809703  UseFilter=on  TunerSelectOption=Transfer Function Based (PID Tuner App)  InitialConditionSource=internal  InitialConditionForIntegrator=0  InitialConditionForFilter=0  DifferentiatorICPrevScaledInput=0  ExternalReset=none  TrackingMode=off  Kt=1  LimitOutput=on  SatLimitsSource=internal  UpperSaturationLimit=.4363  LowerSaturationLimit=-.4363  LinearizeAsGain=off  AntiWindupMode=none  Kb=1  LimitIntegrator=off  UpperIntegratorSaturationLimit=inf  LowerIntegratorSaturationLimit=-inf  POutMin=[]  POutMax=[]  IOutMin=[]  IOutMax=[]  DOutMin=[]  DOutMax=[]  NOutMin=[]  NOutMax=[]  SumOutMin=[]  SumOutMax=[]  SaturationOutMin=[]  SaturationOutMax=[]  PParamMin=[]  PParamMax=[]  IParamMin=[]  IParamMax=[]  DParamMin=[]  DParamMax=[]  NParamMin=[]  NParamMax=[]  KbParamMin=[]  KbParamMax=[]  KtParamMin=[]  KtParamMax=[]  KbOutMin=[]  KbOutMax=[]  KtOutMin=[]  KtOutMax=[]  IntegratorOutMin=[]  IntegratorOutMax=[]  FilterOutMin=[]  FilterOutMax=[]  SumI1OutMin=[]  SumI1OutMax=[]  SumI2OutMin=[]  SumI2OutMax=[]  SumI3OutMin=[]  SumI3OutMax=[]  SumI4OutMin=[]  SumI4OutMax=[]  SumDOutMin=[]  SumDOutMax=[]  DifferentiatorOutMin=[]  DifferentiatorOutMax=[]  FilterDiffOutCoefMin=[]  FilterDiffOutCoefMax=[]  ReciprocalOutMin=[]  ReciprocalOutMax=[]  SumDenOutMin=[]  SumDenOutMax=[]  SumNumOutMin=[]  SumNumOutMax=[]  DivideOutMin=[]  DivideOutMax=[]  UdiffTsProdOutMin=[]  UdiffTsProdOutMax=[]  NTsProdOutMin=[]  NTsProdOutMax=[]  UintegralTsProdOutMin=[]  UintegralTsProdOutMax=[]  UngainTsProdOutMin=[]  UngainTsProdOutMax=[]  ClampingZeroOutDataTypeStr=Inherit: Inherit via back propagation  ClampingZeroOutMin=[]  ClampingZeroOutMax=[]  FilterDenConstantOutDataTypeStr=Inherit: Inherit via back propagation  FilterDenConstantOutMin=[]  FilterDenConstantOutMax=[]  PCopyOutDataTypeStr=Inherit: Inherit via back propagation  PCopyOutMin=[]  PCopyOutMax=[]  NCopyOutDataTypeStr=Inherit: Inherit via back propagation  NCopyOutMin=[]  NCopyOutMax=[]  IntegratorContinuousStateAttributes=''  IntegratorStateMustResolveToSignalObject=off  IntegratorRTWStateStorageClass=Auto  FilterContinuousStateAttributes=''  FilterStateMustResolveToSignalObject=off  FilterRTWStateStorageClass=Auto  ParallelPVariant=InternalParameters  IdealPVariant=Disabled  IVariant=InternalParameters  DVariant=InternalParameters  IntegratorVariant=Continuous  SatVariant=Enabled  AWVariant=Passthrough  PCopyVariant=Disabled  TRVariant=Disabled  FdbkBlocksVariant=Forward  IdealPFdbkVariant=Disabled  SatFdbkVariant=Disabled  DerivativeFilterVariant=ContFilter  NVariant=InternalParameters  NCopyVariant=Disabled  FilterICVariant=InternalICsFilter  IntegratorICVariant=InternalICs  ExternalResetVariant=Disabled  TRSumVariant=Passthrough  SumFdbkVariant=Disabled  SumVariant=Sum_PID  TsampFilterVariant=InternalTs  TsampNgainVariant=Passthrough  TsampIntegralVariant=Disabled_SignalSpec  ExternalSaturationOutDataTypeStr=Inherit: Same as second input  DerivativeSourceVariant=ErrorSignal
  Scope : Scope  Commented=on
  Scope1 : Scope  NumInputPorts=2
  Sum : Sum  Commented=on  Inputs=|+-
  Sum1 : Sum  Inputs=|+-
  Sum2 : Sum  Inputs=|+-
  Terminator{,1..3} (4 alike) : Terminator
  ft/min : Scope  NumInputPorts=2
  del_e_autopilot : Outport
  wires:
  Sum/1 -> Level/1(h_err), If/1  "Error"
  Altitude/1 -> Terminator3/1
  Merge/1 -> ?  "Hal"
  If/1 -> Climb/Action
  If/2 -> Descend/Action
  If/3 -> Level/Action
  Climb/1(del_e_auto) -> Merge/1
  Descend/1(del_e_auto) -> Merge/2
  Level/1(del_e_auto) -> Merge/3
  Merge1/1 -> Scope/1  "Hal"
  Climb/2(Debug) -> Merge1/1
  Descend/2(Debug) -> Merge1/2
  Level/2(Debug) -> Merge1/3
  Input R/C/1 -> Terminator1/1, Terminator/1  "RC"
  Sum1/1 -> Mux/1, Scope1/1  "altitude Error"
  Altitude to ROC commanded/1 -> Sum2/1, Gain/1
  Input R/C1/1 -> Gain1/1, Sum2/2  "RC"
  Sum2/1 -> Scope1/2, PID Controller/1  "ROC error"
  Commanded Altitude1/1 -> Sum1/1
  Altitude1/1 -> Sum1/2
  PID Controller/1 -> del_e_autopilot/1  "Hal"
  Commanded Altitude/1 -> Terminator2/1
  Gain/1 -> ft/min/1  "commanded RC"
  Gain1/1 -> ft/min/2  "RoC"
  Handling/1 -> Mux/2
  Mux/1 -> Altitude to ROC commanded/1

== system Navion_6DoF_10_auto_ascend_2023/Aircraft_Dynamics/Aerodynamics ==
  note: Notes: alpha is measured from
  Wind Para : Inport
  dyn(q) : Inport  Port=2
  Controls : Inport  Port=3
  Mach No. : Inport  Port=4
  a&bdot : Inport  Port=5
  p,q,r : Inport  Port=6
  Aero Forces and Moments : Subsystem
  CD : Subsystem
  CL : Subsystem
  CM : Subsystem
  CN : Subsystem
  CY : Subsystem
  Croll : Subsystem
  Faero : Outport
  Maero : Outport  Port=2
  wires:
  Wind Para/1 -> CY/1(Wind Parameters), Aero Forces and Moments/5(Wind Para), CN/1(Wind Parameters), Croll/1(Wind Parameters), CM/1(Wind Parameters), CD/1(Wind Parameters), CL/1(Wind Parameters)
  CL/1(CL) -> Aero Forces and Moments/4(CL)
  Mach No./1 -> CM/3(Mach No.), CN/3(Mach No.), Croll/3(Mach No.), CY/3(Mach No.), CL/3(Mach No.), CD/3(Mach No.)
  a&bdot/1 -> CL/4(a&bdot), CM/4(a&bdot)
  p,q,r/1 -> CM/5(P,q,r), CN/4(P,q,r), Croll/4(P,q,r), CY/4(P,q,r), CL/5(P,q,r)
  Controls/1 -> CM/2(Controls), CD/2(Controls), CN/2(Controls), Croll/2(Controls), CY/2(Controls), CL/2(Controls)
  CD/1(CD) -> Aero Forces and Moments/2(CD)
  CN/1(CN) -> Aero Forces and Moments/8(CN)
  Croll/1(Croll) -> Aero Forces and Moments/6(Croll)
  CY/1(CY) -> Aero Forces and Moments/3(CY)
  CM/1(CM) -> Aero Forces and Moments/7(CM)
  dyn(q)/1 -> Aero Forces and Moments/1(dyn(q))
  Aero Forces and Moments/1(Faero) -> Faero/1
  Aero Forces and Moments/2(Maero) -> Maero/1

== system Navion_6DoF_10_auto_ascend_2023/Aircraft_Dynamics/Engines ==
  Control : Inport
  Wind Par : Inport  Port=2
  Demux : Demux
  Demux1 : Demux  Outputs=3
  Display : Display
  Max Power : Constant  Value=200*550
  Product : Product  RndMeth=Zero
  Product1 : Product  Inputs=*/  RndMeth=Zero
  Terminator{,1..4} (5 alike) : Terminator
  Feng : Outport
  wires:
  Max Power/1 -> Product/2
  Control/1 -> Demux/1
  Demux/4 -> Product/1
  Demux/1 -> Terminator/1
  Demux/2 -> Terminator1/1
  Demux/3 -> Terminator2/1
  Product/1 -> Product1/1
  Product1/1 -> Feng/1, Display/1
  Wind Par/1 -> Demux1/1
  Demux1/1 -> Product1/2
  Demux1/2 -> Terminator4/1
  Demux1/3 -> Terminator3/1

== system Navion_6DoF_10_auto_ascend_2023/Aircraft_Dynamics/Equations of motion numerical integration  ==
  Accel : Inport
  Inertia : Inport  Port=2
  Moments : Inport  Port=3
  Flat Earth Navigation : Subsystem
  Force Equations : Subsystem
  Gravity Model : Subsystem
  Inert-body : Subsystem
  Kinematic Equiations : Subsystem
  Moment Equations : Subsystem
  Ang Accel : Outport
  Position : Outport  Port=2
  Ang rates : Outport  Port=3
  Wind Vel : Outport  Port=4
  Euler : Outport  Port=5
  R/C : Outport  Port=6
  wires:
  Moment Equations/1(Ang Rates) -> Kinematic Equiations/1(Rates), Force Equations/3(Rates), Ang rates/1
  Kinematic Equiations/1(Euler angles) -> Flat Earth Navigation/1(Euler Angles), Inert-body/1(Euler), Euler/1
  Force Equations/1(Lin Vel) -> Wind Vel/1, Flat Earth Navigation/2(Velocity)
  Accel/1 -> Force Equations/1(Accel)
  Inertia/1 -> Moment Equations/1(Inertia)
  Gravity Model/1(Gravity) -> Force Equations/2(Gravity)
  Moments/1 -> Moment Equations/2(Moments)
  Moment Equations/2(Ang Accel) -> Ang Accel/1
  Flat Earth Navigation/1(Position) -> Position/1
  Inert-body/1(NEDtoBC) -> Force Equations/4(NEDtoABC)
  Flat Earth Navigation/2(R/C) -> R/C/1

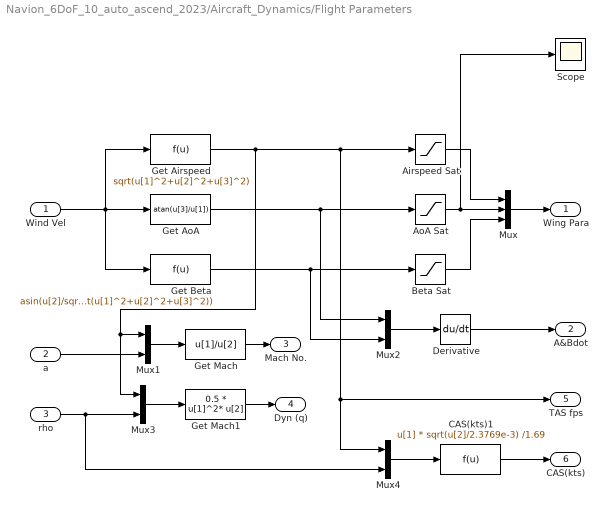
== system Navion_6DoF_10_auto_ascend_2023/Aircraft_Dynamics/Flight Parameters ==
  Wind Vel : Inport
  a : Inport  Port=2
  rho : Inport  Port=3
  Airspeed Sat : Saturate  UpperLimit=1100  LowerLimit=0
  AoA Sat : Saturate  UpperLimit=0.3  LowerLimit=-0.2
  Beta Sat : Saturate  UpperLimit=0.4  LowerLimit=-0.4
  CAS(kts)1 : Fcn  Expr=u[1] * sqrt(u[2]/2.3769e-3) /1.69
  Derivative : Derivative
  Get Airspeed : Fcn  Expr=sqrt(u[1]^2+u[2]^2+u[3]^2)
  Get AoA : Fcn  Expr=atan(u[3]/u[1])
  Get Beta : Fcn  Expr=asin(u[2]/sqrt(u[1]^2+u[2]^2+u[3]^2))
  Get Mach : Fcn  Expr=u[1]/u[2]
  Get Mach1 : Fcn  Expr=0.5 * u[1]^2* u[2]
  Mux : Mux  Inputs=3
  Mux{1..4} (4 alike) : Mux  Inputs=2
  Scope : Scope
  Wing Para : Outport
  A&Bdot : Outport  Port=2
  Mach No. : Outport  Port=3
  Dyn (q) : Outport  Port=4
  TAS fps : Outport  Port=5
  CAS(kts) : Outport  Port=6
  wires:
  Wind Vel/1 -> Get AoA/1, Get Airspeed/1, Get Beta/1
  Get Airspeed/1 -> Mux1/1, Mux3/1, Airspeed Sat/1, TAS fps/1, Mux4/1
  Get AoA/1 -> AoA Sat/1, Mux2/1
  Get Beta/1 -> Beta Sat/1, Mux2/2
  AoA Sat/1 -> Mux/2, Scope/1
  Airspeed Sat/1 -> Mux/1
  Beta Sat/1 -> Mux/3
  Mux/1 -> Wing Para/1
  Mux1/1 -> Get Mach/1
  a/1 -> Mux1/2
  Mux2/1 -> Derivative/1
  Derivative/1 -> A&Bdot/1
  Get Mach/1 -> Mach No./1
  rho/1 -> Mux3/2, Mux4/2
  Mux3/1 -> Get Mach1/1
  Get Mach1/1 -> Dyn (q)/1
  Mux4/1 -> CAS(kts)1/1
  CAS(kts)1/1 -> CAS(kts)/1

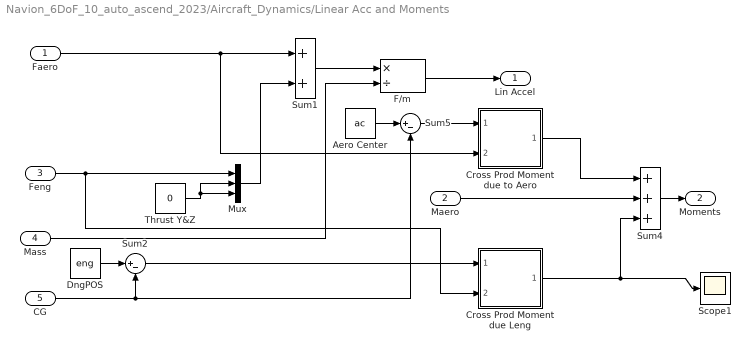
== system Navion_6DoF_10_auto_ascend_2023/Aircraft_Dynamics/Linear Acc and Moments ==
  Faero : Inport
  Maero : Inport  Port=2
  Feng : Inport  Port=3
  Mass : Inport  Port=4
  CG : Inport  Port=5
  Aero Center : Constant  Value=ac
  Cross Prod Moment due Leng : Subsystem
  Cross Prod Moment due to Aero : Subsystem
  DngPOS : Constant  Value=eng
  F/m : Product  Inputs=*/  SaturateOnIntegerOverflow=on  OutDataTypeStr=Inherit: Same as first input
  Mux : Mux  Inputs=3
  Scope1 : Scope
  Sum1 : Sum  SaturateOnIntegerOverflow=on
  Sum2 : Sum  Inputs=|+-  SaturateOnIntegerOverflow=on
  Sum4 : Sum  Inputs=+++  SaturateOnIntegerOverflow=on
  Sum5 : Sum  Inputs=|+-  SaturateOnIntegerOverflow=on
  Thrust Y&Z : Constant  Value=0
  Lin Accel : Outport
  Moments : Outport  Port=2
  wires:
  Feng/1 -> Cross Prod Moment due Leng/2(Vec 2), Mux/1
  Thrust Y&Z/1 -> Mux/2, Mux/3
  Faero/1 -> Sum1/1, Cross Prod Moment due to Aero/2(Vec 2)
  Mux/1 -> Sum1/2
  Sum1/1 -> F/m/1
  Mass/1 -> F/m/2
  F/m/1 -> Lin Accel/1
  CG/1 -> Sum2/2, Sum5/2
  Aero Center/1 -> Sum5/1
  Sum5/1 -> Cross Prod Moment due to Aero/1(Vec 1)
  Maero/1 -> Sum4/2
  Sum4/1 -> Moments/1
  Cross Prod Moment due to Aero/1(X Prod) -> Sum4/1
  Sum2/1 -> Cross Prod Moment due Leng/1(Vec 1)
  Cross Prod Moment due Leng/1(X Prod) -> Sum4/3, Scope1/1
  DngPOS/1 -> Sum2/1

== system Navion_6DoF_10_auto_ascend_2023/Aircraft_Dynamics/Mass, CG & inertia ==
  Mux1 : Mux
  cg : Constant  Value=cg
  jx : Constant  Value=jx
  jxz : Constant  Value=jxz
  jy : Constant  Value=jy
  jz : Constant  Value=jz
  mass2 : Constant  Value=weight/32.2
  CG : Outport
  Inertia : Outport  Port=2
  mass : Outport  Port=3
  wires:
  cg/1 -> CG/1
  jy/1 -> Mux1/2
  jx/1 -> Mux1/1
  jz/1 -> Mux1/3
  jxz/1 -> Mux1/4
  Mux1/1 -> Inertia/1
  mass2/1 -> mass/1

== system Navion_6DoF_10_auto_ascend_2023/Aircraft_Dynamics/Standard Atmosphere ==
  Position : Inport
  Demux : Demux  Outputs=3
      settings: DisplayOption=none
  Density : Fcn  Expr=2.3769e-3*(1 - 0.703e-5 * u[1])^4.14
  OATemp : Lookup  InputValues=[0 35000 60000]  Table=[519 390 390]
  Speed of Sound : Fcn  Expr=sqrt(1.4*1716.3*u[1])
  Terminator : Terminator
  Terminator1 : Terminator
  OAT : Outport
  rho : Outport  Port=2
  a : Outport  Port=3
  Hp : Outport  Port=4
  wires:
  OATemp/1 -> OAT/1, Speed of Sound/1
  Density/1 -> rho/1
  Speed of Sound/1 -> a/1
  Position/1 -> Demux/1
  Demux/1 -> Terminator/1
  Demux/2 -> Terminator1/1
  Demux/3 -> OATemp/1, Density/1, Hp/1

== system Navion_6DoF_10_auto_ascend_2023/Bank Angle PID/roll ==
  In1 : Inport
  Demux : Demux  Outputs=3
  Terminator : Terminator
  Terminator1 : Terminator
  Out1 : Outport
  wires:
  In1/1 -> Demux/1
  Demux/2 -> Terminator/1
  Demux/3 -> Terminator1/1
  Demux/1 -> Out1/1

== system Navion_6DoF_10_auto_ascend_2023/longitudinal autopilot/Climb ==
  note: this is desired rate of climb
  note: the PID gains different because it has a different input, its not altitude but rate of climb
  R/C : Inport
  Action Port : ActionPort  ActionPortLabel=if(u1 > 100)
  Debugging : Constant
  Fcn : Fcn  Expr=u(1)/60
  PID Controller : slpidlib/PID Controller  Controller=PID  Form=Parallel  TimeDomain=Continuous-time  UseExternalTs=off  SampleTime=-1  IntegratorMethod=Forward Euler  FilterMethod=Forward Euler  ControllerParametersSource=internal  P=1  I=1  UseKiTs=off  D=0  N=100  UseFilter=on  TunerSelectOption=Transfer Function Based (PID Tuner App)  InitialConditionSource=internal  InitialConditionForIntegrator=0  InitialConditionForFilter=0  DifferentiatorICPrevScaledInput=0  ExternalReset=none  TrackingMode=off  Kt=1  LimitOutput=off  SatLimitsSource=internal  UpperSaturationLimit=inf  LowerSaturationLimit=-inf  LinearizeAsGain=on  AntiWindupMode=none  Kb=1  LimitIntegrator=off  UpperIntegratorSaturationLimit=inf  LowerIntegratorSaturationLimit=-inf  POutMin=[]  POutMax=[]  IOutMin=[]  IOutMax=[]  DOutMin=[]  DOutMax=[]  NOutMin=[]  NOutMax=[]  SumOutMin=[]  SumOutMax=[]  SaturationOutMin=[]  SaturationOutMax=[]  PParamMin=[]  PParamMax=[]  IParamMin=[]  IParamMax=[]  DParamMin=[]  DParamMax=[]  NParamMin=[]  NParamMax=[]  KbParamMin=[]  KbParamMax=[]  KtParamMin=[]  KtParamMax=[]  KbOutMin=[]  KbOutMax=[]  KtOutMin=[]  KtOutMax=[]  IntegratorOutMin=[]  IntegratorOutMax=[]  FilterOutMin=[]  FilterOutMax=[]  SumI1OutMin=[]  SumI1OutMax=[]  SumI2OutMin=[]  SumI2OutMax=[]  SumI3OutMin=[]  SumI3OutMax=[]  SumI4OutMin=[]  SumI4OutMax=[]  SumDOutMin=[]  SumDOutMax=[]  DifferentiatorOutMin=[]  DifferentiatorOutMax=[]  FilterDiffOutCoefMin=[]  FilterDiffOutCoefMax=[]  ReciprocalOutMin=[]  ReciprocalOutMax=[]  SumDenOutMin=[]  SumDenOutMax=[]  SumNumOutMin=[]  SumNumOutMax=[]  DivideOutMin=[]  DivideOutMax=[]  UdiffTsProdOutMin=[]  UdiffTsProdOutMax=[]  NTsProdOutMin=[]  NTsProdOutMax=[]  UintegralTsProdOutMin=[]  UintegralTsProdOutMax=[]  UngainTsProdOutMin=[]  UngainTsProdOutMax=[]  ClampingZeroOutDataTypeStr=Inherit: Inherit via back propagation  ClampingZeroOutMin=[]  ClampingZeroOutMax=[]  FilterDenConstantOutDataTypeStr=Inherit: Inherit via back propagation  FilterDenConstantOutMin=[]  FilterDenConstantOutMax=[]  PCopyOutDataTypeStr=Inherit: Inherit via back propagation  PCopyOutMin=[]  PCopyOutMax=[]  NCopyOutDataTypeStr=Inherit: Inherit via back propagation  NCopyOutMin=[]  NCopyOutMax=[]  IntegratorContinuousStateAttributes=''  IntegratorStateMustResolveToSignalObject=off  IntegratorRTWStateStorageClass=Auto  FilterContinuousStateAttributes=''  FilterStateMustResolveToSignalObject=off  FilterRTWStateStorageClass=Auto  ParallelPVariant=InternalParameters  IdealPVariant=Disabled  IVariant=InternalParameters  DVariant=InternalParameters  IntegratorVariant=Continuous  SatVariant=Disabled  AWVariant=Passthrough  PCopyVariant=Disabled  TRVariant=Disabled  FdbkBlocksVariant=Forward  IdealPFdbkVariant=Disabled  SatFdbkVariant=Disabled  DerivativeFilterVariant=ContFilter  NVariant=InternalParameters  NCopyVariant=Disabled  FilterICVariant=InternalICsFilter  IntegratorICVariant=InternalICs  ExternalResetVariant=Disabled  TRSumVariant=Passthrough  SumFdbkVariant=Disabled  SumVariant=Sum_PID  TsampFilterVariant=InternalTs  TsampNgainVariant=Passthrough  TsampIntegralVariant=Disabled_SignalSpec  ExternalSaturationOutDataTypeStr=Inherit: Same as second input
  R/C_CMD : Constant  Value=1000
  Sum : Sum  Inputs=|+-
  del_e_auto : Outport
  Debug : Outport  Port=2
  wires:
  R/C/1 -> Sum/1
  PID Controller/1 -> del_e_auto/1
  Sum/1 -> PID Controller/1
  R/C_CMD/1 -> Fcn/1
  Debugging/1 -> Debug/1
  Fcn/1 -> Sum/2
